simulink model "parte4_eje4_Tvapor160223"  (R2019b)
settings: Solver=VariableStepAuto  StartTime=0.0  StopTime=10.0  RelTol=1e-3
values from neighbouring files (symbols this model uses):
  FHP = 0.3    [parte4_eje2_TVapor.m]
  FIP = 0.3    [parte4_eje2_TVapor.m]
  FLP = 0.4    [parte4_eje2_TVapor.m]
  TCH = 0.3    [parte4_eje2_TVapor.m]
  TCO = 0.5    [parte4_eje2_TVapor.m]
  TRH = 7    [parte4_eje2_TVapor.m]
settings Model: Creator=cjuar  LastModifiedBy=cjuar

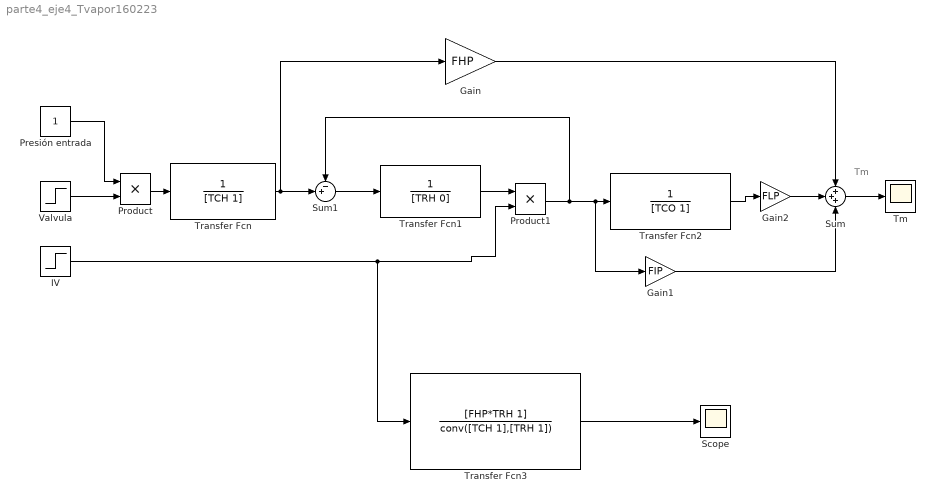
== system parte4_eje4_Tvapor160223 ==
  note: Tm
  Gain : Gain  Gain=FHP
  Gain1 : Gain  Gain=FIP
  Gain2 : Gain  Gain=FLP
  "IV " : Step  SampleTime=0
  Presión entrada : Constant
  Product : Product
  Product1 : Product
  Scope : Scope
  Sum : Sum  Inputs=+++
  Sum1 : Sum  Inputs=-+|
  Tm : Scope
  Transfer Fcn : TransferFcn  Denominator=[TCH 1]
  Transfer Fcn1 : TransferFcn  Denominator=[TRH 0]
  Transfer Fcn2 : TransferFcn  Denominator=[TCO 1]
  Transfer Fcn3 : TransferFcn  Numerator=[FHP*TRH 1]  Denominator=conv([TCH 1],[TRH 1])
  "Valvula " : Step  SampleTime=0
  wires:
  Presión entrada/1 -> Product/1
  "Valvula "/1 -> Product/2
  Product/1 -> Transfer Fcn/1
  Transfer Fcn/1 -> Sum1/2, Gain/1
  Transfer Fcn1/1 -> Product1/1
  "IV "/1 -> Product1/2, Transfer Fcn3/1
  Product1/1 -> Sum1/1, Transfer Fcn2/1, Gain1/1
  Gain/1 -> Sum/1
  Sum/1 -> Tm/1
  Gain1/1 -> Sum/3
  Sum1/1 -> Transfer Fcn1/1
  Gain2/1 -> Sum/2
  Transfer Fcn2/1 -> Gain2/1
  Transfer Fcn3/1 -> Scope/1
